simulink model "ysw3_26"  (Simulink 8.3)
settings: Solver=ode4  StartTime=0.0  StopTime=2  RelTol=1e-3
settings Model: Creator=hp  LastModifiedBy=Administrator  ExtModeTrigMode=oneshot  ExtModeArmWhenConnect=off
settings DataIOCC: Decimation=100  LimitDataPoints=off  SaveOutput=off  SaveTime=off
settings OptimizationCC: BlockReduction=off  BooleanDataType=off  InitFltsAndDblsToZero=on
settings DebuggingCC: SaveWithParameterizedLinksMsg=none  SignalResolutionControl=TryResolveAllWithWarning  SolverPrmCheckMsg=none  MultiTaskDSMMsg=warning  MultiTaskCondExecSysMsg=none  FcnCallInpInsideContextMsg=UseLocalSettings  StateNameClashWarn=none
settings HardwareCC: TargetUnknown=on
settings RTWCC: IncludeERTFirstTime=on
settings GRTTargetCC: TargetFcnLib=ansi_tfl_tmw.mat

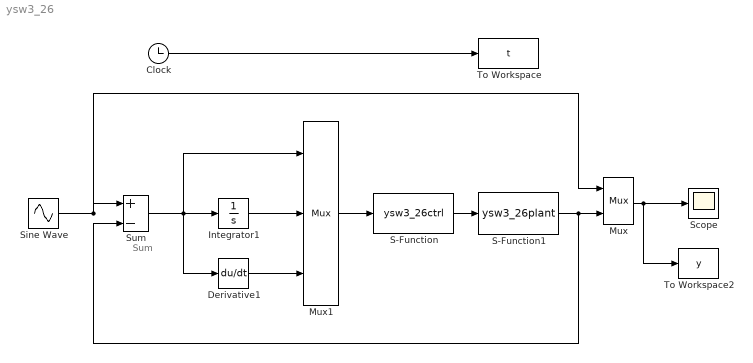
== system ysw3_26 ==
  note: Sum
  Clock : Clock
  Derivative1 : Derivative
  Integrator1 : Integrator
  Mux : Mux  Inputs=2
  Mux1 : Mux  Inputs=3
  S-Function : S-Function  FunctionName=ysw3_26ctrl  EnableBusSupport=off
  S-Function1 : S-Function  FunctionName=ysw3_26plant  EnableBusSupport=off
  Scope : Scope
      settings: TimeRange=0.2  YMin=-0.051  YMax=-0.041  MaxDataPoints=50000  Decimation=0.001  SampleInput=on  SampleTime=0.001
  Sine Wave : Sin  Amplitude=0.50  Frequency=1*2*pi  SampleTime=0
  Sum : Sum  Inputs=|+-  SaturateOnIntegerOverflow=on  InputSameDT=on  OutDataTypeStr=Inherit: Same as first input
  To Workspace : ToWorkspace  VariableName=t  SampleTime=-1
  To Workspace2 : ToWorkspace  VariableName=y  SampleTime=-1
  wires:
  Mux/1 -> Scope/1, To Workspace2/1
  S-Function/1 -> S-Function1/1
  Mux1/1 -> S-Function/1
  Sine Wave/1 -> Sum/1, Mux/1
  Derivative1/1 -> Mux1/3
  Integrator1/1 -> Mux1/2
  Sum/1 -> Integrator1/1, Derivative1/1, Mux1/1
  S-Function1/1 -> Mux/2, Sum/2
  Clock/1 -> To Workspace/1
